simulink model "matlab_simulink"  (R2025a)
settings: Solver=VariableStepAuto  StartTime=0.0  StopTime=10.0  RelTol=1e-3
libraries: arduinolib x4, simulink x2
settings Model: SimulationMode=accelerator

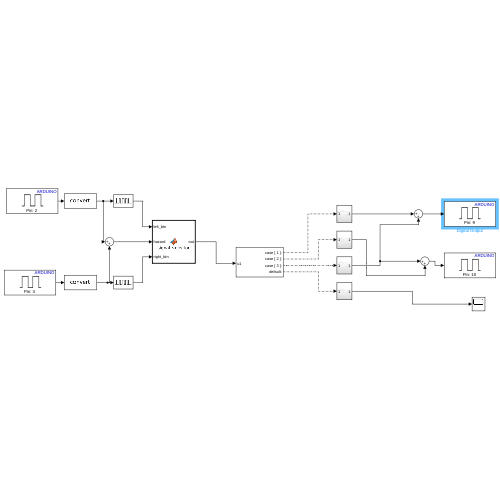
[thumbnail: Simulink's stored preview of the top-level diagram]
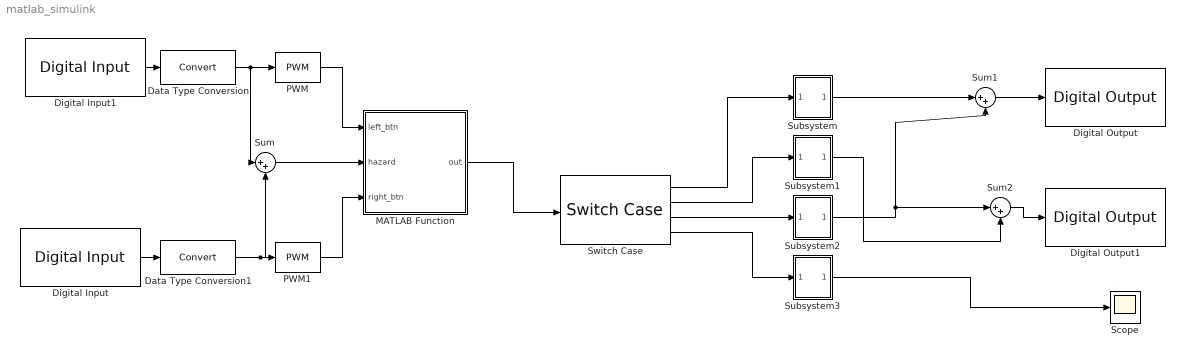
== system matlab_simulink ==
  Data Type Conversion : DataTypeConversion  SaturateOnIntegerOverflow=off  RndMeth=Floor
  Data Type Conversion1 : DataTypeConversion  SaturateOnIntegerOverflow=off  RndMeth=Floor
  Digital Input : arduinolib/Digital Input  pinNumber=3  mode=Input Pullup  Direction=input  SampleTime=0.1  blockPlatform=arduino
  Digital Input1 : arduinolib/Digital Input  pinNumber=2  mode=Input Pullup  Direction=input  SampleTime=0.1  blockPlatform=arduino
  Digital Output : arduinolib/Digital Output  pinNumber=9  Direction=output  blockPlatform=arduino
  Digital Output1 : arduinolib/Digital Output  pinNumber=10  Direction=output  blockPlatform=arduino
  MATLAB Function : MATLAB Function  TreatAsAtomicUnit=on
  PWM : simulink/Discontinuities/PWM  DisableCoverage=on  Period=1  InitialDelay=0  DisallowZeroDutyCycle=off  RunAtFixedTimeIntervals=off  SampleTime=0.1
  PWM1 : simulink/Discontinuities/PWM  DisableCoverage=on  Period=1  InitialDelay=0  DisallowZeroDutyCycle=off  RunAtFixedTimeIntervals=off  SampleTime=0.1
  Scope : Scope
      settings: ActiveDisplayYMinimum=-0.12499999999999997  ActiveDisplayYMaximum=1.125
  Subsystem : Subsystem
  Subsystem1 : Subsystem
  Subsystem2 : Subsystem
  Subsystem3 : Subsystem
  Sum : Sum  Inputs=|++
  Sum1 : Sum  Inputs=|++
  Sum2 : Sum  Inputs=|++
  Switch Case : SwitchCase  CaseConditions={1,2,3}
  wires:
  MATLAB Function/1(out) -> Switch Case/1
  Switch Case/1 -> Subsystem/1(In1)
  Subsystem/1(Out1) -> Sum1/1
  Switch Case/2 -> Subsystem1/1(In1)
  Switch Case/3 -> Subsystem2/1(In1)
  Subsystem2/1(Out1) -> Sum2/1, Sum1/2
  Subsystem3/1(Out1) -> Scope/1
  Switch Case/4 -> Subsystem3/1(In1)
  Sum/1 -> MATLAB Function/2(hazard)
  PWM/1 -> MATLAB Function/1(left_btn)
  Subsystem1/1(Out1) -> Sum2/2
  Sum2/1 -> Digital Output1/1
  Sum1/1 -> Digital Output/1
  Digital Input1/1 -> Data Type Conversion/1
  Digital Input/1 -> Data Type Conversion1/1
  Data Type Conversion1/1 -> Sum/2, PWM1/1
  PWM1/1 -> MATLAB Function/3(right_btn)
  Data Type Conversion/1 -> Sum/1, PWM/1

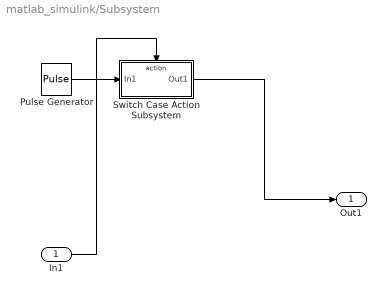
== system matlab_simulink/Subsystem ==
  In1 : Inport
  Pulse Generator : DiscretePulseGenerator  PulseType=Time based  Period=1  PulseWidth=30
  Switch Case Action Subsystem : Subsystem  TreatAsAtomicUnit=on
  Out1 : Outport
  wires:
  Pulse Generator/1 -> Switch Case Action Subsystem/1(In1)
  In1/1 -> Switch Case Action Subsystem/Action
  Switch Case Action Subsystem/1(Out1) -> Out1/1

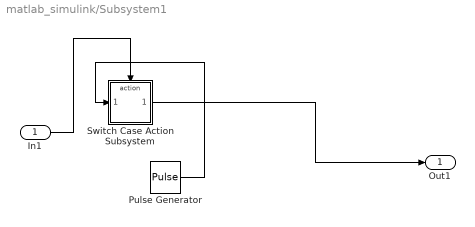
== system matlab_simulink/Subsystem1 ==
  In1 : Inport
  Pulse Generator : DiscretePulseGenerator  PulseType=Time based  Period=1  PulseWidth=30
  Switch Case Action Subsystem : Subsystem  TreatAsAtomicUnit=on
  Out1 : Outport
  wires:
  Pulse Generator/1 -> Switch Case Action Subsystem/1(In1)
  Switch Case Action Subsystem/1(Out1) -> Out1/1
  In1/1 -> Switch Case Action Subsystem/Action

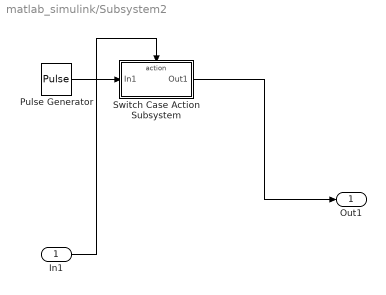
== system matlab_simulink/Subsystem2 ==
  In1 : Inport
  Pulse Generator : DiscretePulseGenerator  PulseType=Time based  Period=1  PulseWidth=30
  Switch Case Action Subsystem : Subsystem  TreatAsAtomicUnit=on
  Out1 : Outport
  wires:
  Pulse Generator/1 -> Switch Case Action Subsystem/1(In1)
  In1/1 -> Switch Case Action Subsystem/Action
  Switch Case Action Subsystem/1(Out1) -> Out1/1

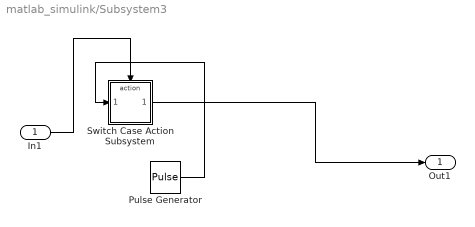
== system matlab_simulink/Subsystem3 ==
  In1 : Inport
  Pulse Generator : DiscretePulseGenerator  PulseType=Time based  Period=1  PulseWidth=30
  Switch Case Action Subsystem : Subsystem  TreatAsAtomicUnit=on
  Out1 : Outport
  wires:
  Pulse Generator/1 -> Switch Case Action Subsystem/1(In1)
  Switch Case Action Subsystem/1(Out1) -> Out1/1
  In1/1 -> Switch Case Action Subsystem/Action

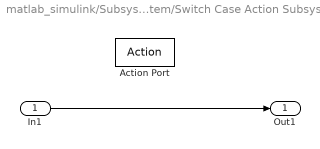
== system matlab_simulink/Subsystem/Switch Case Action Subsystem ==
  In1 : Inport
  Action Port : ActionPort  ActionPortLabel=case [ 1 ]:
  Out1 : Outport
  wires:
  In1/1 -> Out1/1

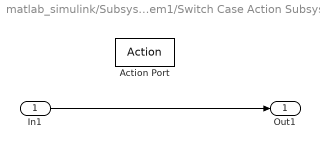
== system matlab_simulink/Subsystem1/Switch Case Action Subsystem ==
  In1 : Inport
  Action Port : ActionPort  ActionPortLabel=case [ 2 ]:
  Out1 : Outport
  wires:
  In1/1 -> Out1/1

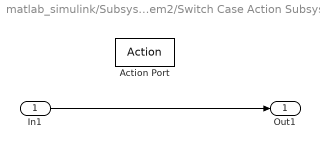
== system matlab_simulink/Subsystem2/Switch Case Action Subsystem ==
  In1 : Inport
  Action Port : ActionPort  ActionPortLabel=case [ 3 ]:
  Out1 : Outport
  wires:
  In1/1 -> Out1/1

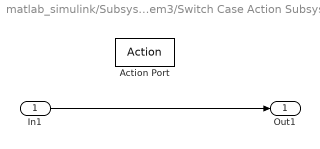
== system matlab_simulink/Subsystem3/Switch Case Action Subsystem ==
  In1 : Inport
  Action Port : ActionPort  ActionPortLabel=default:
  Out1 : Outport
  wires:
  In1/1 -> Out1/1

== matlab function matlab_simulink/MATLAB Function ==
  data: left_btn input; out output; hazard input; right_btn input
function out = signal_selector( left_btn,hazard, right_btn)
    if left_btn == 1
        out = 1;
    elseif hazard == 1
        out = 2;
    elseif right_btn == 1
        out = 3;
    else
        out = 0;
    end
end
